simulink model "Project_UR5"  (Simulink 8.3)
settings: Solver=ode3  StartTime=0.0  StopTime=tf  FixedStep=ts  RelTol=1e-3
values from neighbouring files (symbols this model uses):
  qi = [0;pi/4;0;-pi/3;0;0]    [initial.m]
(part 3 of 3)

== matlab function Trajectory Planning ==
  data: t input double; des output double
function des = TRJ(t)
%% %% Geometric Path
%% Rectilinear Path
% Pi = [-500 100 600].';
% Pf = [ 200 200 800].';
% L = norm(Pf-Pi);

%%Don't Uncomment
%x_des = Pi + s*(Pf - Pi)/L;
%xd_des = (Pf-Pi)*sd/L;

%% Circlar Path 
r = 150 ;        %Circle Radius
O = [-200 -100 700].' ; %Center
L = 2*pi*r ;    %for circular path
di = [1 1 0].' ; %Direction Vector of the circle Plane
ndi = norm(di) ; di = di/ndi ; %Normalizing di vector

if di(1) == 0 && di(2) == 0
    R = eye(3); % no rotaion
else
a = asin(di(2)/(sqrt((di(1))^2+(di(2))^2))) ; %Roation around Z
b = acos(di(3));                              %Roation around y
Ra = [cos(a) -sin(a)   0;
      sin(a)  cos(a)  0;
        0      0      1];
    
Rb = [cos(b)  0   sin(b);
        0     1     0   ;
     -sin(b)  0  cos(b)];
 
R = Ra*Rb ;
end

% %%Don't Uncomment
%x_des = O + R*[r*cos(s/r) r*sin(s/r) 0].' ;
%xd_des = R*[-sin(s/r) cos(s/r) 0].' ;

%% %% Timing Law
s = 0;
sd = 0;

T = 4.9; % tf = T
T_s = T/8;
vmax = L/(T-T_s);
amax = vmax/T_s;

if t<=T_s
    s = amax*t^2/2;
    sd = amax*t;
elseif t>T_s && t<T-T_s
    s = vmax*t - vmax^2/(2*amax);
    sd = vmax;
elseif t>=T-T_s && t<=T
    s = -amax*(t-T)^2/2 + vmax*T - vmax^2/amax;
    sd = vmax - amax*(t-T+T_s);
end

%% Commands x_des xd_des based on path
%%Circular Path
% x_des = O + R*[r*cos(s/r) r*sin(s/r) 0].' ;
% xd_des = R*[-sin(s/r) cos(s/r) 0].' ;

%%Helix Path
w = 2000;
x_des = O + R*[r*cos(w*t/r) r*sin(w*t/r) 50*t].' ;
xd_des = R*[-w*sin(w*t/r) w*cos(w*t/r) 25].' ;

%%Rectilinear Path
% x_des = Pi + s*(Pf - Pi)/L;
% xd_des = (Pf-Pi)*sd/L;

%%No timing law line_Test
% x_des=[100+50*t 200 400].' ;
% xd_des=[50 0 0].' ;

des=[x_des;xd_des];

== matlab function  Task Error ==
  data: x_des input double; q input double; err output double
function err = Error(x_des,q)

%Input Decomposition
q1 = q(1);
q2 = q(2);
q3 = q(3);
q4 = q(4);
q5 = q(5);
q6 = q(6);

%% End effector Position
x = [(379*cos(q2 + q3)*cos(q1)*sin(q4))/4 - 425*cos(q1)*cos(q2) - (165*cos(q5)*sin(q1))/2 - (165*cos(q2 + q3 + q4)*cos(q1)*sin(q5))/2 - (1093*sin(q1))/10 + (379*sin(q2 + q3)*cos(q1)*cos(q4))/4 - 392*cos(q1)*cos(q2)*cos(q3) + 392*cos(q1)*sin(q2)*sin(q3);
(1093*cos(q1))/10 + (165*cos(q1)*cos(q5))/2 - 425*cos(q2)*sin(q1) + 392*sin(q1)*sin(q2)*sin(q3) - (165*cos(q2 + q3 + q4)*sin(q1)*sin(q5))/2 + (379*cos(q2 + q3)*sin(q1)*sin(q4))/4 + (379*sin(q2 + q3)*cos(q4)*sin(q1))/4 - 392*cos(q2)*cos(q3)*sin(q1);
392*sin(q2 + q3) + 425*sin(q2) + sin(q5)*((165*cos(q2 + q3)*sin(q4))/2 + (165*sin(q2 + q3)*cos(q4))/2) + (379*cos(q2 + q3)*cos(q4))/4 - (379*sin(q2 + q3)*sin(q4))/4 + 446/5];

%% Error Calulation
e = x_des-x;
err = norm(e);
